simulink library "xbsDSP48_r3"  (Simulink 5.0)
libraries: xbsIndex_r3 x429, xbsDSP48_r3 x2
(part 5 of 8)

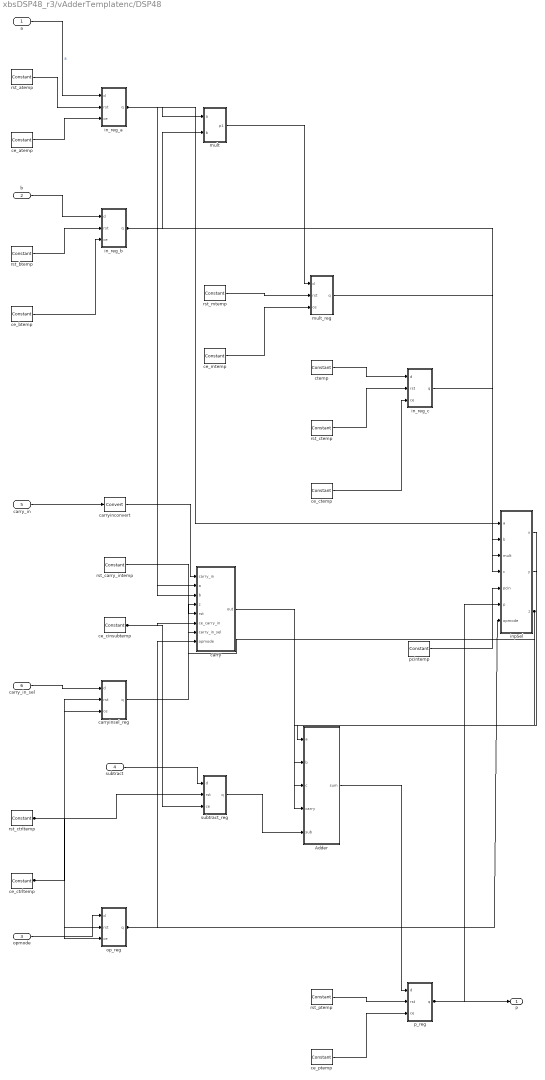
== system xbsDSP48_r3/vAdderTemplatenc/DSP48 ==
  a : Inport
  b : Inport  Port=2
  opmode : Inport  Port=3
  subtract : Inport  Port=4
  carry_in : Inport  Port=5
  carry_in_sel : Inport  Port=6
  Adder : Subsystem
  carry : Subsystem
  carryinconvert : xbsIndex_r3/Convert  arith_type=Unsigned  n_bits=1  bin_pt=0  quantization=Truncate  overflow=Wrap  latency=0  explicit_period=off  period=1  dbl_ovrd=off  show_param=off  inserted_by_tool=off  pipeline=off
      settings: xl_area=[0, 0, 0, 0, 0, 0, 0]
  carryinsel_reg : Subsystem  mask{nreg=pipeline_carryinsel, pnreg=1}
      mask prompts: nreg "Number of registers"; pnreg "Previous number of register"
      mask init: same as xbsDSP48_r3/DSP48reg
      mask Display:
      | patch([0 iWidth iWidth 0],[0 0 iHeight iHeight] , bg);
      | patch(logoX,logoY , fg);
      | text(iCx-6,iCy,'z');
      | text(iCx,iCy+4,str);
      | port_label('input',1,'d');
      | port_label('input',2,'rst');
      | port_label('input',3,'ce');
      | port_label('output',1,'q');
      | plot([0 0 iWidth iWidth 0], [0 iHeight iHeight 0 0]);
  ce_atemp : xbsIndex_r3/Constant  const=1  equ=P=C  arith_type=Boolean  n_bits=1  bin_pt=0  opselect=C  inp2=PCIN>>17  opr=+  inp1=P  carry=CIN  iostate=0  explicit_period=on  period=1  dbl_ovrd=off
  ce_btemp : xbsIndex_r3/Constant  const=1  equ=P=C  arith_type=Boolean  n_bits=1  bin_pt=0  opselect=C  inp2=PCIN>>17  opr=+  inp1=P  carry=CIN  iostate=0  explicit_period=on  period=1  dbl_ovrd=off
  ce_cinsubtemp : xbsIndex_r3/Constant  const=1  equ=P=C  arith_type=Boolean  n_bits=1  bin_pt=0  opselect=C  inp2=PCIN>>17  opr=+  inp1=P  carry=CIN  iostate=0  explicit_period=on  period=1  dbl_ovrd=off
  ce_ctemp : xbsIndex_r3/Constant  const=1  equ=P=C  arith_type=Boolean  n_bits=1  bin_pt=0  opselect=C  inp2=PCIN>>17  opr=+  inp1=P  carry=CIN  iostate=0  explicit_period=on  period=1  dbl_ovrd=off
  ce_ctrltemp : xbsIndex_r3/Constant  const=1  equ=P=C  arith_type=Boolean  n_bits=1  bin_pt=0  opselect=C  inp2=PCIN>>17  opr=+  inp1=P  carry=CIN  iostate=0  explicit_period=on  period=1  dbl_ovrd=off
  ce_mtemp : xbsIndex_r3/Constant  const=1  equ=P=C  arith_type=Boolean  n_bits=1  bin_pt=0  opselect=C  inp2=PCIN>>17  opr=+  inp1=P  carry=CIN  iostate=0  explicit_period=on  period=1  dbl_ovrd=off
  ce_ptemp : xbsIndex_r3/Constant  const=1  equ=P=C  arith_type=Boolean  n_bits=1  bin_pt=0  opselect=C  inp2=PCIN>>17  opr=+  inp1=P  carry=CIN  iostate=0  explicit_period=on  period=1  dbl_ovrd=off
  ctemp : xbsIndex_r3/Constant  const=1  equ=P=C  arith_type="Signed  (2's comp)"  n_bits=48  bin_pt=0  opselect=C  inp2=PCIN>>17  opr=+  inp1=P  carry=CIN  iostate=0  explicit_period=on  period=1  dbl_ovrd=off
  in_reg_a : Subsystem  mask{nreg=pipeline_a-1, pnreg=1}
      mask prompts: nreg "Number of registers"; pnreg "Previous number of register"
      mask init: same as xbsDSP48_r3/DSP48reg
      mask Display:
      | patch([0 iWidth iWidth 0],[0 0 iHeight iHeight] , bg);
      | patch(logoX,logoY , fg);
      | text(iCx-6,iCy,'z');
      | text(iCx,iCy+4,str);
      | port_label('input',1,'d');
      | port_label('input',2,'rst');
      | port_label('input',3,'ce');
      | port_label('output',1,'q');
      | plot([0 0 iWidth iWidth 0], [0 iHeight iHeight 0 0]);
  in_reg_b : Subsystem  mask{nreg=pipeline_b- 1, pnreg=1}
      mask prompts: nreg "Number of registers"; pnreg "Previous number of register"
      mask init: same as xbsDSP48_r3/DSP48reg
      mask Display:
      | patch([0 iWidth iWidth 0],[0 0 iHeight iHeight] , bg);
      | patch(logoX,logoY , fg);
      | text(iCx-6,iCy,'z');
      | text(iCx,iCy+4,str);
      | port_label('input',1,'d');
      | port_label('input',2,'rst');
      | port_label('input',3,'ce');
      | port_label('output',1,'q');
      | plot([0 0 iWidth iWidth 0], [0 iHeight iHeight 0 0]);
  in_reg_c : Subsystem  mask{nreg=pipeline_c, pnreg=1}
      mask prompts: nreg "Number of registers"; pnreg "Previous number of register"
      mask init: same as xbsDSP48_r3/DSP48reg
      mask Display:
      | patch([0 iWidth iWidth 0],[0 0 iHeight iHeight] , bg);
      | patch(logoX,logoY , fg);
      | text(iCx-6,iCy,'z');
      | text(iCx,iCy+4,str);
      | port_label('input',1,'d');
      | port_label('input',2,'rst');
      | port_label('input',3,'ce');
      | port_label('output',1,'q');
      | plot([0 0 iWidth iWidth 0], [0 iHeight iHeight 0 0]);
  inpSel : Subsystem
  mult : Subsystem
  mult_reg : Subsystem  mask{nreg=pipeline_mult, pnreg=1}
      mask prompts: nreg "Number of registers"; pnreg "Previous number of register"
      mask init: same as xbsDSP48_r3/DSP48reg
      mask Display:
      | patch([0 iWidth iWidth 0],[0 0 iHeight iHeight] , bg);
      | patch(logoX,logoY , fg);
      | text(iCx-6,iCy,'z');
      | text(iCx,iCy+4,str);
      | port_label('input',1,'d');
      | port_label('input',2,'rst');
      | port_label('input',3,'ce');
      | port_label('output',1,'q');
      | plot([0 0 iWidth iWidth 0], [0 iHeight iHeight 0 0]);
  op_reg : Subsystem  mask{nreg=pipeline_opmode, pnreg=1}
      mask prompts: nreg "Number of registers"; pnreg "Previous number of register"
      mask init: same as xbsDSP48_r3/DSP48reg
      mask Display:
      | patch([0 iWidth iWidth 0],[0 0 iHeight iHeight] , bg);
      | patch(logoX,logoY , fg);
      | text(iCx-6,iCy,'z');
      | text(iCx,iCy+4,str);
      | port_label('input',1,'d');
      | port_label('input',2,'rst');
      | port_label('input',3,'ce');
      | port_label('output',1,'q');
      | plot([0 0 iWidth iWidth 0], [0 iHeight iHeight 0 0]);
  p_reg : Subsystem  mask{nreg=pipeline_p, pnreg=1}
      mask prompts: nreg "Number of registers"; pnreg "Previous number of register"
      mask init: same as xbsDSP48_r3/DSP48reg
      mask Display:
      | patch([0 iWidth iWidth 0],[0 0 iHeight iHeight] , bg);
      | patch(logoX,logoY , fg);
      | text(iCx-6,iCy,'z');
      | text(iCx,iCy+4,str);
      | port_label('input',1,'d');
      | port_label('input',2,'rst');
      | port_label('input',3,'ce');
      | port_label('output',1,'q');
      | plot([0 0 iWidth iWidth 0], [0 iHeight iHeight 0 0]);
  pcintemp : xbsIndex_r3/Constant  const=1  equ=P=C  arith_type="Signed  (2's comp)"  n_bits=48  bin_pt=0  opselect=C  inp2=PCIN>>17  opr=+  inp1=P  carry=CIN  iostate=0  explicit_period=on  period=1  dbl_ovrd=off
  rst_atemp : xbsIndex_r3/Constant  const=0  equ=P=C  arith_type=Boolean  n_bits=1  bin_pt=0  opselect=C  inp2=PCIN>>17  opr=+  inp1=P  carry=CIN  iostate=0  explicit_period=on  period=1  dbl_ovrd=off
  rst_btemp : xbsIndex_r3/Constant  const=0  equ=P=C  arith_type=Boolean  n_bits=1  bin_pt=0  opselect=C  inp2=PCIN>>17  opr=+  inp1=P  carry=CIN  iostate=0  explicit_period=on  period=1  dbl_ovrd=off
  rst_carry_intemp : xbsIndex_r3/Constant  const=0  equ=P=C  arith_type=Boolean  n_bits=1  bin_pt=0  opselect=C  inp2=PCIN>>17  opr=+  inp1=P  carry=CIN  iostate=0  explicit_period=on  period=1  dbl_ovrd=off
  rst_ctemp : xbsIndex_r3/Constant  const=0  equ=P=C  arith_type=Boolean  n_bits=1  bin_pt=0  opselect=C  inp2=PCIN>>17  opr=+  inp1=P  carry=CIN  iostate=0  explicit_period=on  period=1  dbl_ovrd=off
  rst_ctrltemp : xbsIndex_r3/Constant  const=0  equ=P=C  arith_type=Boolean  n_bits=1  bin_pt=0  opselect=C  inp2=PCIN>>17  opr=+  inp1=P  carry=CIN  iostate=0  explicit_period=on  period=1  dbl_ovrd=off
  rst_mtemp : xbsIndex_r3/Constant  const=0  equ=P=C  arith_type=Boolean  n_bits=1  bin_pt=0  opselect=C  inp2=PCIN>>17  opr=+  inp1=P  carry=CIN  iostate=0  explicit_period=on  period=1  dbl_ovrd=off
  rst_ptemp : xbsIndex_r3/Constant  const=0  equ=P=C  arith_type=Boolean  n_bits=1  bin_pt=0  opselect=C  inp2=PCIN>>17  opr=+  inp1=P  carry=CIN  iostate=0  explicit_period=on  period=1  dbl_ovrd=off
  subtract_reg : Subsystem  mask{nreg=pipeline_sub, pnreg=1}
      mask prompts: nreg "Number of registers"; pnreg "Previous number of register"
      mask init: same as xbsDSP48_r3/DSP48reg
      mask Display:
      | patch([0 iWidth iWidth 0],[0 0 iHeight iHeight] , bg);
      | patch(logoX,logoY , fg);
      | text(iCx-6,iCy,'z');
      | text(iCx,iCy+4,str);
      | port_label('input',1,'d');
      | port_label('input',2,'rst');
      | port_label('input',3,'ce');
      | port_label('output',1,'q');
      | plot([0 0 iWidth iWidth 0], [0 iHeight iHeight 0 0]);
  P : Outport
  wires:
  ce_cinsubtemp/1 -> subtract_reg/3(ce), carry/6(ce_carry_in)
  ce_ctrltemp/1 -> op_reg/3(ce), carryinsel_reg/3(ce)
  rst_ctrltemp/1 -> carryinsel_reg/2(rst), subtract_reg/2(rst), op_reg/2(rst)
  p_reg/1(q) -> inpSel/6(p), P/1
  in_reg_b/1(q) -> carry/3(b), inpSel/2(b), mult/2(b)
  op_reg/1(q) -> carry/8(opmode), inpSel/7(opmode)
  inpSel/3(z) -> carry/4(z), Adder/3(c)
  in_reg_a/1(q) -> inpSel/1(a), carry/2(a), mult/1(a)
  ctemp/1 -> in_reg_c/1(d)
  pcintemp/1 -> inpSel/5(pcin)
  ce_mtemp/1 -> mult_reg/3(ce)
  ce_ptemp/1 -> p_reg/3(ce)
  ce_ctemp/1 -> in_reg_c/3(ce)
  ce_btemp/1 -> in_reg_b/3(ce)
  ce_atemp/1 -> in_reg_a/3(ce)
  rst_carry_intemp/1 -> carry/5(rst)
  rst_mtemp/1 -> mult_reg/2(rst)
  rst_ptemp/1 -> p_reg/2(rst)
  rst_ctemp/1 -> in_reg_c/2(rst)
  rst_btemp/1 -> in_reg_b/2(rst)
  rst_atemp/1 -> in_reg_a/2(rst)
  b/1 -> in_reg_b/1(d)
  carryinsel_reg/1(q) -> carry/7(carry_in_sel)
  carry_in_sel/1 -> carryinsel_reg/1(d)
  carry_in/1 -> carryinconvert/1
  opmode/1 -> op_reg/1(d)
  a/1 -> in_reg_a/1(d)  "a"
  subtract/1 -> subtract_reg/1(d)
  carry/1(out) -> Adder/4(carry)
  subtract_reg/1(q) -> Adder/5(sub)
  Adder/1(sum) -> p_reg/1(d)
  inpSel/2(y) -> Adder/2(b)
  inpSel/1(x) -> Adder/1(a)
  mult_reg/1(q) -> inpSel/3(mult)
  mult/1(p1) -> mult_reg/1(d)
  in_reg_c/1(q) -> inpSel/4(c)
  carryinconvert/1 -> carry/1(carry_in)

== system xbsDSP48_r3/vDSP48/Adder ==
  a : Inport
  b : Inport  Port=2
  c : Inport  Port=3
  carry : Inport  Port=4
  sub : Inport  Port=5
  Add1 : xbsIndex_r3/AddSub  mode=Addition  precision=User Defined  arith_type="Signed  (2's comp)"  n_bits=48  bin_pt=0  quantization=Truncate  overflow=Wrap  latency=0  explicit_period=off  period=1  use_carryin=off  use_carryout=off  en=off  dbl_ovrd=off  show_param=off  use_core=on  pipeline=off  use_rpm=off  gen_core=on
      settings: xl_area=[0, 0, 0, 0, 0, 0, 0]
  AddSub : xbsIndex_r3/AddSub  mode=Addition or Subtraction  precision=User Defined  arith_type="Signed  (2's comp)"  n_bits=48  bin_pt=0  quantization=Truncate  overflow=Wrap  latency=0  explicit_period=on  period=period  use_carryin=off  use_carryout=off  en=off  dbl_ovrd=off  show_param=off  use_core=on  pipeline=off  use_rpm=off  gen_core=on
      settings: xl_area=[0, 0, 0, 0, 0, 0, 0]
  AddSub1 : xbsIndex_r3/AddSub  mode=Addition  precision=User Defined  arith_type="Signed  (2's comp)"  n_bits=48  bin_pt=0  quantization=Truncate  overflow=Wrap  latency=0  explicit_period=off  period=1  use_carryin=off  use_carryout=off  en=off  dbl_ovrd=off  show_param=off  use_core=on  pipeline=off  use_rpm=off  gen_core=on
      settings: xl_area=[0, 0, 0, 0, 0, 0, 0]
  Convert : xbsIndex_r3/Convert  arith_type=Boolean  n_bits=8  bin_pt=6  quantization=Truncate  overflow=Wrap  latency=0  explicit_period=off  period=1  dbl_ovrd=off  show_param=off  inserted_by_tool=off  pipeline=off
      settings: xl_area=[0, 0, 0, 0, 0, 0, 0]
  sum : Outport
  wires:
  a/1 -> Add1/1
  b/1 -> Add1/2
  AddSub/1 -> sum/1
  sub/1 -> Convert/1
  Convert/1 -> AddSub/3
  carry/1 -> AddSub1/2
  c/1 -> AddSub/1
  Add1/1 -> AddSub1/1
  AddSub1/1 -> AddSub/2

== system xbsDSP48_r3/vDSP48/carry ==
  carry_in : Inport
  a : Inport  Port=2
  b : Inport  Port=3
  z : Inport  Port=4
  rst : Inport  Port=5
  ce_carry_in : Inport  Port=6
  carry_in_sel : Inport  Port=7
  opmode : Inport  Port=8
  Convert : xbsIndex_r3/Convert  arith_type=Boolean  n_bits=8  bin_pt=6  quantization=Truncate  overflow=Wrap  latency=0  explicit_period=off  period=1  dbl_ovrd=off  show_param=off  inserted_by_tool=off  pipeline=off
      settings: xl_area=[0, 0, 0, 0, 0, 0, 0]
  Convert2 : xbsIndex_r3/Convert  arith_type=Boolean  n_bits=8  bin_pt=6  quantization=Truncate  overflow=Wrap  latency=0  explicit_period=off  period=1  dbl_ovrd=off  show_param=off  inserted_by_tool=off  pipeline=off
      settings: xl_area=[0, 0, 0, 0, 0, 0, 0]
  Inverter : xbsIndex_r3/Inverter  latency=0  explicit_period=off  period=1  en=off  dbl_ovrd=off  show_param=off
      settings: xl_area=[0, 0, 0, 0, 0, 0, 0]
  Inverter1 : xbsIndex_r3/Inverter  latency=0  explicit_period=off  period=1  en=off  dbl_ovrd=off  show_param=off
      settings: xl_area=[0, 0, 0, 0, 0, 0, 0]
  Logical : xbsIndex_r3/Logical  logical_function=XNOR  inputs=2  precision=User Defined  arith_type=Unsigned  n_bits=1  bin_pt=0  align_bp=on  latency=0  explicit_period=off  period=1  en=off  dbl_ovrd=off  show_param=off
      settings: xl_area=[0, 0, 0, 0, 0, 0, 0]
  Mux : xbsIndex_r3/Mux  inputs=4  precision=User Defined  arith_type=Unsigned  n_bits=1  bin_pt=0  quantization=Truncate  overflow=Wrap  latency=0  explicit_period=off  period=1  en=off  dbl_ovrd=off  show_param=off  mux_type=off  use_rpm=off  gen_core=on
      settings: xl_area=[0, 0, 0, 0, 0, 0, 0]
  Mux1 : xbsIndex_r3/Mux  inputs=2  precision=User Defined  arith_type=Unsigned  n_bits=1  bin_pt=0  quantization=Truncate  overflow=Wrap  latency=0  explicit_period=off  period=1  en=off  dbl_ovrd=off  show_param=off  mux_type=off  use_rpm=off  gen_core=on
      settings: xl_area=[0, 0, 0, 0, 0, 0, 0]
  Register2 : xbsIndex_r3/Register  init=0  reg_only_valid=off  explicit_period=off  period=1  rst=on  en=on  out_en=off  dbl_ovrd=off  show_param=off
      settings: xl_area=[0, 0, 0, 0, 0, 0, 0]
  Slice : xbsIndex_r3/Slice  mode=Lower Bit Location + Width  nbits=1  bit1=17  base1=MSB of Input  bit0=17  base0=LSB of Input  boolean_output=off  explicit_period=off  period=1  dbl_ovrd=off
  Slice1 : xbsIndex_r3/Slice  mode=Lower Bit Location + Width  nbits=1  bit1=17  base1=MSB of Input  bit0=17  base0=LSB of Input  boolean_output=off  explicit_period=off  period=1  dbl_ovrd=off
  Slice2 : xbsIndex_r3/Slice  mode=Lower Bit Location + Width  nbits=1  bit1=17  base1=MSB of Input  bit0=6  base0=LSB of Input  boolean_output=off  explicit_period=off  period=1  dbl_ovrd=off
  Slice3 : xbsIndex_r3/Slice  mode=Lower Bit Location + Width  nbits=1  bit1=17  base1=MSB of Input  bit0=47  base0=LSB of Input  boolean_output=off  explicit_period=off  period=1  dbl_ovrd=off
  carryin_reg : Subsystem  mask{nreg=pipeline_carryin, pnreg=1}
      mask prompts: nreg "Number of registers"; pnreg "Previous number of register"
      mask init: same as xbsDSP48_r3/DSP48reg
      mask Display:
      | patch([0 iWidth iWidth 0],[0 0 iHeight iHeight] , bg);
      | patch(logoX,logoY , fg);
      | text(iCx-6,iCy,'z');
      | text(iCx,iCy+4,str);
      | port_label('input',1,'d');
      | port_label('input',2,'rst');
      | port_label('input',3,'ce');
      | port_label('output',1,'q');
      | plot([0 0 iWidth iWidth 0], [0 iHeight iHeight 0 0]);
  out : Outport
  wires:
  carry_in/1 -> carryin_reg/1(d)
  Slice3/1 -> Inverter1/1
  Slice2/1 -> Mux1/1
  Inverter1/1 -> Mux/3  "z47"
  Convert2/1 -> Register2/2, carryin_reg/2(rst)
  Convert/1 -> Register2/3
  Logical/1 -> Mux1/3
  Slice1/1 -> Logical/2
  Slice/1 -> Inverter/1, Logical/1
  Inverter/1 -> Mux1/2
  b/1 -> Slice1/1
  a/1 -> Slice/1
  z/1 -> Slice3/1
  Register2/1 -> Mux/5  "carryreg"
  carryin_reg/1(q) -> Mux/2  "carryin"
  ce_carry_in/1 -> Convert/1, carryin_reg/3(ce)
  Mux1/1 -> Mux/4, Register2/1  "carrybyp"
  carry_in_sel/1 -> Mux/1
  Mux/1 -> out/1
  rst/1 -> Convert2/1
  opmode/1 -> Slice2/1

== system xbsDSP48_r3/vDSP48/carryinsel_reg ==
  d : Inport
  rst : Inport  Port=2
  ce : Inport  Port=3
  Register1 : xbsIndex_r3/Register  init=0  reg_only_valid=off  explicit_period=off  period=1  rst=on  en=on  out_en=off  dbl_ovrd=off  show_param=off
      settings: xl_area=[0, 0, 0, 0, 0, 0, 0]
  q : Outport
  wires:
  d/1 -> Register1/1
  rst/1 -> Register1/2
  ce/1 -> Register1/3
  Register1/1 -> q/1

== system xbsDSP48_r3/vDSP48/in_reg_a ==
  d : Inport
  rst : Inport  Port=2
  ce : Inport  Port=3
  Register1 : xbsIndex_r3/Register  init=0  reg_only_valid=off  explicit_period=off  period=1  rst=on  en=on  out_en=off  dbl_ovrd=off  show_param=off
      settings: xl_area=[0, 0, 0, 0, 0, 0, 0]
  q : Outport
  wires:
  d/1 -> Register1/1
  rst/1 -> Register1/2
  ce/1 -> Register1/3
  Register1/1 -> q/1

== system xbsDSP48_r3/vDSP48/in_reg_b ==
  d : Inport
  rst : Inport  Port=2
  ce : Inport  Port=3
  Register1 : xbsIndex_r3/Register  init=0  reg_only_valid=off  explicit_period=off  period=1  rst=on  en=on  out_en=off  dbl_ovrd=off  show_param=off
      settings: xl_area=[0, 0, 0, 0, 0, 0, 0]
  q : Outport
  wires:
  d/1 -> Register1/1
  rst/1 -> Register1/2
  ce/1 -> Register1/3
  Register1/1 -> q/1

== system xbsDSP48_r3/vDSP48/in_reg_c ==
  d : Inport
  rst : Inport  Port=2
  ce : Inport  Port=3
  Register1 : xbsIndex_r3/Register  init=0  reg_only_valid=off  explicit_period=off  period=1  rst=on  en=on  out_en=off  dbl_ovrd=off  show_param=off
      settings: xl_area=[0, 0, 0, 0, 0, 0, 0]
  q : Outport
  wires:
  d/1 -> Register1/1
  rst/1 -> Register1/2
  ce/1 -> Register1/3
  Register1/1 -> q/1

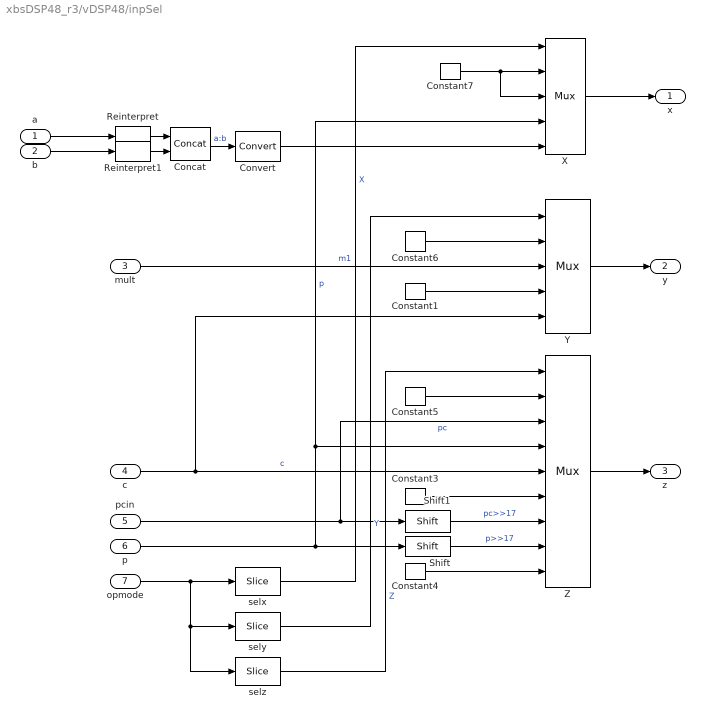
== system xbsDSP48_r3/vDSP48/inpSel ==
  a : Inport
  b : Inport  Port=2
  mult : Inport  Port=3
  c : Inport  Port=4
  pcin : Inport  Port=5
  p : Inport  Port=6
  opmode : Inport  Port=7
  Concat : xbsIndex_r3/Concat  num_inputs=2  explicit_period=off  period=1  dbl_ovrd=off
  Constant{1,3..7} (6 alike) : xbsIndex_r3/Constant  const=0  equ=P=C  arith_type="Signed  (2's comp)"  n_bits=48  bin_pt=0  opselect=C  inp2=PCIN>>17  opr=+  inp1=P  carry=CIN  iostate=0  explicit_period=off  period=1  dbl_ovrd=off
  Convert : xbsIndex_r3/Convert  arith_type="Signed  (2's comp)"  n_bits=36  bin_pt=0  quantization=Truncate  overflow=Wrap  latency=0  explicit_period=off  period=1  dbl_ovrd=off  show_param=off  inserted_by_tool=off  pipeline=off
      settings: xl_area=[0, 0, 0, 0, 0, 0, 0]
  Reinterpret : xbsIndex_r3/Reinterpret  force_arith_type=on  arith_type=Unsigned  force_bin_pt=on  bin_pt=0  force_valid=on
  Reinterpret1 : xbsIndex_r3/Reinterpret  force_arith_type=on  arith_type=Unsigned  force_bin_pt=on  bin_pt=0  force_valid=on
  Shift : xbsIndex_r3/Shift  shift_dir=Right  shift_bits=17  precision=Full  arith_type="Signed  (2's comp)"  n_bits=8  bin_pt=2  quantization=Truncate  overflow=Wrap  latency=0  explicit_period=off  period=1  en=off  dbl_ovrd=off  show_param=off
      settings: xl_area=[0, 0, 0, 0, 0, 0, 0]
  Shift1 : xbsIndex_r3/Shift  shift_dir=Right  shift_bits=17  precision=Full  arith_type="Signed  (2's comp)"  n_bits=8  bin_pt=2  quantization=Truncate  overflow=Wrap  latency=0  explicit_period=off  period=1  en=off  dbl_ovrd=off  show_param=off
      settings: xl_area=[0, 0, 0, 0, 0, 0, 0]
  X : xbsIndex_r3/Mux  inputs=4  precision=User Defined  arith_type="Signed  (2's comp)"  n_bits=48  bin_pt=0  quantization=Truncate  overflow=Wrap  latency=0  explicit_period=off  period=1  en=off  dbl_ovrd=off  show_param=off  mux_type=off  use_rpm=off  gen_core=on
      settings: xl_area=[0, 0, 0, 0, 0, 0, 0]
  Y : xbsIndex_r3/Mux  inputs=4  precision=User Defined  arith_type="Signed  (2's comp)"  n_bits=48  bin_pt=0  quantization=Truncate  overflow=Wrap  latency=0  explicit_period=off  period=1  en=off  dbl_ovrd=off  show_param=off  mux_type=off  use_rpm=off  gen_core=on
      settings: xl_area=[0, 0, 0, 0, 0, 0, 0]
  Z : xbsIndex_r3/Mux  inputs=8  precision=User Defined  arith_type="Signed  (2's comp)"  n_bits=48  bin_pt=0  quantization=Truncate  overflow=Wrap  latency=0  explicit_period=off  period=1  en=off  dbl_ovrd=off  show_param=off  mux_type=off  use_rpm=off  gen_core=on
      settings: xl_area=[0, 0, 0, 0, 0, 0, 0]
  selx : xbsIndex_r3/Slice  mode=Lower Bit Location + Width  nbits=2  bit1=0  base1=MSB of Input  bit0=0  base0=LSB of Input  boolean_output=off  explicit_period=off  period=1  dbl_ovrd=off
  sely : xbsIndex_r3/Slice  mode=Lower Bit Location + Width  nbits=2  bit1=2  base1=MSB of Input  bit0=2  base0=LSB of Input  boolean_output=off  explicit_period=off  period=1  dbl_ovrd=off
  selz : xbsIndex_r3/Slice  mode=Lower Bit Location + Width  nbits=3  bit1=0  base1=MSB of Input  bit0=4  base0=LSB of Input  boolean_output=off  explicit_period=off  period=1  dbl_ovrd=off
  x : Outport
  y : Outport  Port=2
  z : Outport  Port=3
  wires:
  Reinterpret1/1 -> Concat/2
  Reinterpret/1 -> Concat/1
  sely/1 -> Y/1  "Y"
  selx/1 -> X/1  "X"
  mult/1 -> Y/3  "m1"
  c/1 -> Z/5, Y/5  "c"
  Constant7/1 -> X/3, X/2
  Constant6/1 -> Y/2
  Constant5/1 -> Z/2
  Constant3/1 -> Z/6
  Shift/1 -> Z/8  "p>>17"
  Shift1/1 -> Z/7  "pc>>17"
  Constant4/1 -> Z/9
  Constant1/1 -> Y/4
  selz/1 -> Z/1  "Z"
  opmode/1 -> sely/1, selz/1, selx/1
  p/1 -> Z/4, X/4, Shift/1  "p"
  Z/1 -> z/1
  Y/1 -> y/1
  X/1 -> x/1
  b/1 -> Reinterpret1/1
  a/1 -> Reinterpret/1
  Concat/1 -> Convert/1  "a:b"
  pcin/1 -> Z/3, Shift1/1  "pc"
  Convert/1 -> X/5

== system xbsDSP48_r3/vDSP48/mult ==
  a : Inport
  b : Inport  Port=2
  Mult : xbsIndex_r3/Mult  precision=User Defined  arith_type="Signed  (2's comp)"  n_bits=36  bin_pt=0  quantization=Truncate  overflow=Wrap  latency=0  explicit_period=off  period=1  en=off  dbl_ovrd=off  show_param=on  mult_type=Parallel  oversample=2  use_embedded=on  pipeline=off  use_rpm=off  placement_style=Rectangular Shape  gen_core=on
      settings: xl_area=[0, 0, 0, 0, 0, 0, 0]
  p1 : Outport
  wires:
  b/1 -> Mult/2
  a/1 -> Mult/1
  Mult/1 -> p1/1

== system xbsDSP48_r3/vDSP48/mult_reg ==
  d : Inport
  rst : Inport  Port=2
  ce : Inport  Port=3
  Register1 : xbsIndex_r3/Register  init=0  reg_only_valid=off  explicit_period=off  period=1  rst=on  en=on  out_en=off  dbl_ovrd=off  show_param=off
      settings: xl_area=[0, 0, 0, 0, 0, 0, 0]
  q : Outport
  wires:
  d/1 -> Register1/1
  rst/1 -> Register1/2
  ce/1 -> Register1/3
  Register1/1 -> q/1

== system xbsDSP48_r3/vDSP48/op_reg ==
  d : Inport
  rst : Inport  Port=2
  ce : Inport  Port=3
  Register1 : xbsIndex_r3/Register  init=0  reg_only_valid=off  explicit_period=off  period=1  rst=on  en=on  out_en=off  dbl_ovrd=off  show_param=off
      settings: xl_area=[0, 0, 0, 0, 0, 0, 0]
  q : Outport
  wires:
  d/1 -> Register1/1
  rst/1 -> Register1/2
  ce/1 -> Register1/3
  Register1/1 -> q/1

== system xbsDSP48_r3/vDSP48/p_reg ==
  d : Inport
  rst : Inport  Port=2
  ce : Inport  Port=3
  Register1 : xbsIndex_r3/Register  init=0  reg_only_valid=off  explicit_period=off  period=1  rst=on  en=on  out_en=off  dbl_ovrd=off  show_param=off
      settings: xl_area=[0, 0, 0, 0, 0, 0, 0]
  q : Outport
  wires:
  d/1 -> Register1/1
  rst/1 -> Register1/2
  ce/1 -> Register1/3
  Register1/1 -> q/1

== system xbsDSP48_r3/vDSP48/subtract_reg ==
  d : Inport
  rst : Inport  Port=2
  ce : Inport  Port=3
  Register1 : xbsIndex_r3/Register  init=0  reg_only_valid=off  explicit_period=off  period=1  rst=on  en=on  out_en=off  dbl_ovrd=off  show_param=off
      settings: xl_area=[0, 0, 0, 0, 0, 0, 0]
  q : Outport
  wires:
  d/1 -> Register1/1
  rst/1 -> Register1/2
  ce/1 -> Register1/3
  Register1/1 -> q/1
